simulink model "mdlObstacle"  (Simulink 8.6)
settings: Solver=ode5  StartTime=0.0  StopTime=tmax  FixedStep=0.0001  MaxStep=1e-2  RelTol=1e-4
values from neighbouring files (symbols this model uses):
  delta = 0.1    [settings.m]
  doutside = 0    [settings.m]
  emax = 0.08    [settings.m]
  gradoutside = 10    [settings.m]
  k2 = 0    [settings.m]
  r1 = 1    [settings.m]
  r2 = 0    [settings.m]
  x1t = 3    [settings.m]
  x2t = 0    [settings.m]
settings Model: Creator=rsanfelice  LastModifiedBy=Vijay  ExtModeAutoUpdateStatusClock=off
settings DataIOCC: SaveOutput=off  SaveTime=off  SignalLoggingName=sigsOut
settings OptimizationCC: BooleanDataType=off  ExpressionDepthLimit=128  InitFltsAndDblsToZero=on
settings DebuggingCC: SaveWithParameterizedLinksMsg=none  SignalResolutionControl=TryResolveAllWithWarning  SolverPrmCheckMsg=none  MultiTaskDSMMsg=warning  MultiTaskCondExecSysMsg=none  FcnCallInpInsideContextMsg=UseLocalSettings  StateNameClashWarn=none
settings HardwareCC: TargetUnknown=on
settings GRTTargetCC: TargetFcnLib=ansi_tfl_tmw.mat  GeneratePreprocessorConditionals=Use local settings

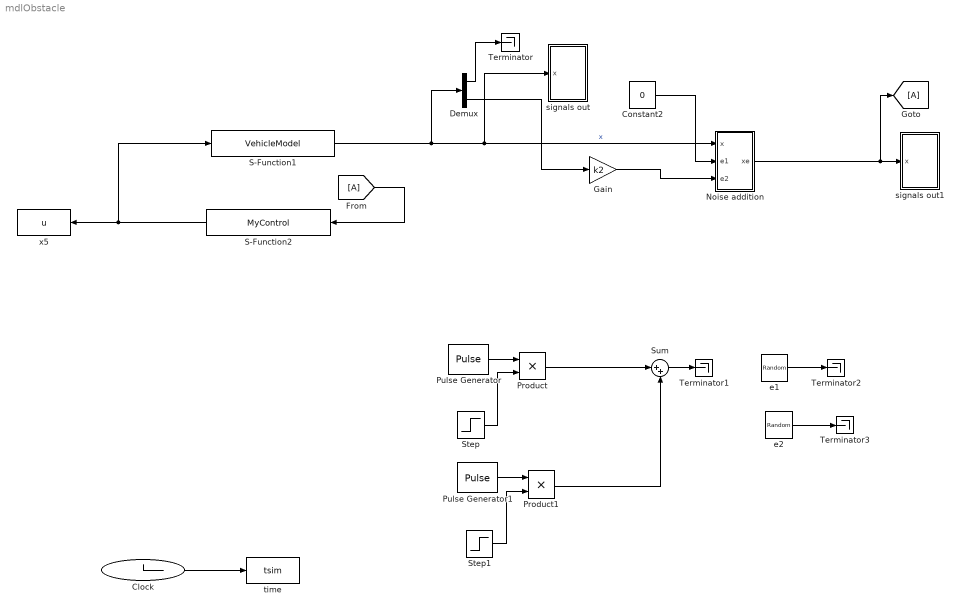
== system mdlObstacle ==
  Clock : Clock
  Constant2 : Constant  Value=0
  Demux : Demux  Outputs=2
  Gain : Gain  Gain=k2
  Noise addition : Subsystem
  Product : Product  RndMeth=Zero
  Product1 : Product  RndMeth=Zero
  Pulse Generator : DiscretePulseGenerator  PulseType=Time based  Amplitude=emax  Period=0.005  PulseWidth=50
  Pulse Generator1 : DiscretePulseGenerator  PulseType=Time based  Amplitude=-emax  Period=0.005  PulseWidth=50
  S-Function1 : S-Function  FunctionName=VehicleModel  Parameters=x0  SFunctionDeploymentMode=off  EnableBusSupport=off
  S-Function2 : S-Function  FunctionName=MyControl  Parameters=0,r1,r2,delta,gradoutside,doutside,x1t,x2t  SFunctionDeploymentMode=off  EnableBusSupport=off
  Step : Step  Time=0.04  Before=1  After=0  SampleTime=0
  Step1 : Step  Time=0.04  SampleTime=0
  Sum : Sum  Inputs=|++
  Terminator{,1..3} (4 alike) : Terminator
  e1 : RandomNumber  Variance=1*emax  SampleTime=0
  e2 : RandomNumber  Variance=1*emax  SampleTime=0
  signals out : Subsystem
  signals out1 : Subsystem
  time : ToWorkspace  VariableName=tsim  SampleTime=-1
  x5 : ToWorkspace  VariableName=u  SampleTime=-1
  wires:
  Clock/1 -> time/1
  S-Function1/1 -> signals out/1(x), Noise addition/1(x), Demux/1  "x"
  S-Function2/1 -> x5/1, S-Function1/1
  Noise addition/1(xe) -> signals out1/1(x), [A]
  [A] -> S-Function2/1
  Pulse Generator/1 -> Product/1
  Step/1 -> Product/2
  Product/1 -> Sum/1
  Pulse Generator1/1 -> Product1/1
  Step1/1 -> Product1/2
  Product1/1 -> Sum/2
  Constant2/1 -> Noise addition/2(e1)
  Gain/1 -> Noise addition/3(e2)
  Demux/2 -> Gain/1
  Demux/1 -> Terminator/1
  Sum/1 -> Terminator1/1
  e1/1 -> Terminator2/1
  e2/1 -> Terminator3/1

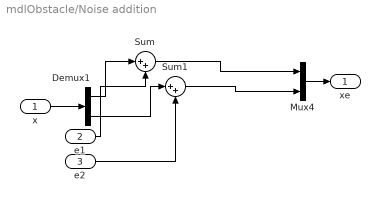
== system mdlObstacle/Noise addition ==
  x : Inport
  e1 : Inport  Port=2
  e2 : Inport  Port=3
  Demux1 : Demux  Outputs=2
  Mux4 : Mux  Inputs=2
  Sum : Sum  Inputs=|++
  Sum1 : Sum  Inputs=|++
  xe : Outport
  wires:
  Demux1/1 -> Sum/1
  Demux1/2 -> Sum1/1
  Sum/1 -> Mux4/1
  Sum1/1 -> Mux4/2
  x/1 -> Demux1/1
  Mux4/1 -> xe/1
  e1/1 -> Sum/2
  e2/1 -> Sum1/2

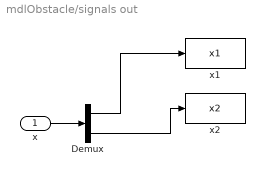
== system mdlObstacle/signals out ==
  x : Inport
  Demux : Demux  Outputs=2
  x1 : ToWorkspace  VariableName=x1  SampleTime=-1
  x2 : ToWorkspace  VariableName=x2  SampleTime=-1
  wires:
  Demux/1 -> x1/1
  Demux/2 -> x2/1
  x/1 -> Demux/1

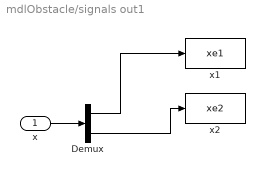
== system mdlObstacle/signals out1 ==
  x : Inport
  Demux : Demux  Outputs=2
  x1 : ToWorkspace  VariableName=xe1  SampleTime=-1
  x2 : ToWorkspace  VariableName=xe2  SampleTime=-1
  wires:
  Demux/1 -> x1/1
  Demux/2 -> x2/1
  x/1 -> Demux/1
